simulink model "EvitarObstaculo"  (R2023b)
settings: Solver=FixedStepAuto  StartTime=0.0  StopTime=100  FixedStep=Ts  RelTol=1e-3
values from neighbouring files (symbols this model uses):
  obsx = 2    [TryOut.m]
  obsy = 0.5    [TryOut.m]
  refx = 5    [TryOut.m]
  refy = 5    [TryOut.m]
  Ts = 100e-3    (= 0.1)    [TryOut.m]
undefined symbols (not defined in the file or in its folder): DiscIntNeverNeededParam, sigbuilder_block, th_0, x_0, y_0
libraries: fuzblock x1
settings Model: Creator=Francisco  LastModifiedBy=Francisco
settings DataIOCC: ReturnWorkspaceOutputs=off

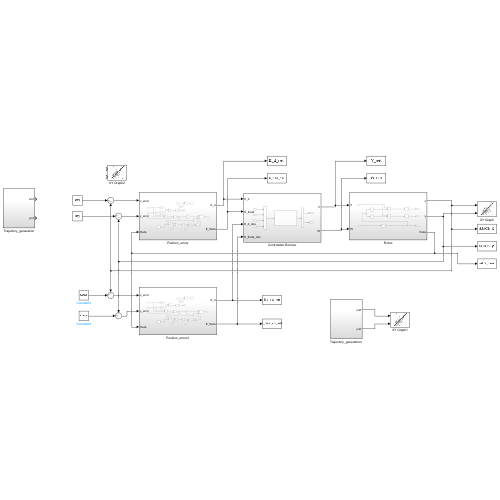
[thumbnail: Simulink's stored preview of the top-level diagram]
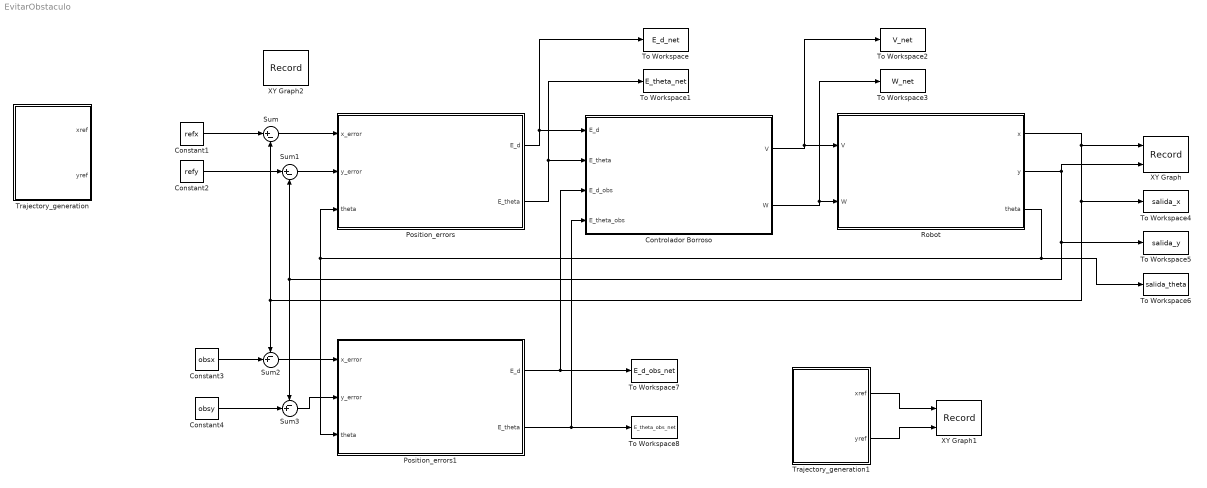
== system EvitarObstaculo ==
  Constant1 : Constant  Value=refx
  Constant2 : Constant  Value=refy
  Constant3 : Constant  Value=obsx
  Constant4 : Constant  Value=obsy
  Controlador Borroso : Subsystem
  Position_errors : Subsystem
  Position_errors1 : Subsystem
  Robot : Subsystem
  Sum : Sum  Inputs=|+-
  Sum1 : Sum  Inputs=|+-
  Sum2 : Sum  Inputs=-+|
  Sum3 : Sum  Inputs=-+|
  To Workspace : ToWorkspace  VariableName=E_d_net  SaveFormat=Structure With Time  SampleTime=-1
  To Workspace1 : ToWorkspace  VariableName=E_theta_net  SaveFormat=Structure With Time  SampleTime=-1
  To Workspace2 : ToWorkspace  VariableName=V_net  SaveFormat=Structure With Time  SampleTime=-1
  To Workspace3 : ToWorkspace  VariableName=W_net  SaveFormat=Structure With Time  SampleTime=-1
  To Workspace4 : ToWorkspace  VariableName=salida_x  SaveFormat=Structure With Time  SampleTime=-1
  To Workspace5 : ToWorkspace  VariableName=salida_y  SaveFormat=Structure With Time  SampleTime=-1
  To Workspace6 : ToWorkspace  VariableName=salida_theta  SaveFormat=Structure With Time  SampleTime=-1
  To Workspace7 : ToWorkspace  VariableName=E_d_obs_net  SaveFormat=Structure With Time  SampleTime=-1
  To Workspace8 : ToWorkspace  VariableName=E_theta_obs_net  SaveFormat=Structure With Time  SampleTime=-1
  Trajectory_generation : Subsystem
  Trajectory_generation1 : Subsystem
  XY Graph : Record  FileSettingsInternal="{\"entries\":[{\"content\":{\"excelSettings\":{\"content\":{},\"type\":\"Streamout.ExcelSettings\"}},\"type\":\"Streamout.FileSettingStorage\",\"uuid\":\"\"}],\"packageUris\":[\"http:\\/\\/schema.mathworks.com\\/mf0\\/streamout_blocks\\/R2020a\"],\"version\":\"1.0\"}"  Layout=[1 1]  SignalsInternal="{\"entries\":[{\"content\":{\"signals\":[{\"content\":{\"blockPath\":[],\"dimensions\":[1],\"domain\":\"\",\"lineColor\":\"#0072bd\",\"plots\":[1],\"port\":1,\"sid\":[\"\"],\"signalID\":8880,\"signalName\":\"Robot:1\"},\"type\":\"RecordBlkView.Signal\",\"uuid\":\"\"},{\"content\":{\"blockPath\":[],\"dimensions\":[1],\"domain\":\"\",\"lineColor\":\"#d95319\",\"plots\":[1],\"port\":2,\"sid\":[\"\"],\"signalID\":8884,\"signalName\":\"Robot:2\"},\"type\":\"RecordBlkView.Signal\",\"uuid\":\"\"}]},\"type\":\"RecordBlkView.InputSignals\",\"uuid\":\"\"}],\"packageUris\":[\"http:\\/\\/schema.mathworks.com\\/mf0\\/streamout_blocks\\/R2020a\"],\"version\":\"1.0\"}"  VisualizationBindings="{\"xyplotplugin\":{\"info\":[{\"series\":[{\"bindingParametersList\":[{\"parameter\":\"X-Axis\",\"signalID\":8880,\"signalName\":\"Robot:1\"},{\"parameter\":\"Y-Axis\",\"signalID\":8884,\"signalName\":\"Robot:2\"}],\"seriesID\":59230}],\"subplotID\":1}]}}"  CompatibilityTag=XY
  XY Graph1 : Record  FileSettingsInternal="{\"entries\":[{\"content\":{\"excelSettings\":{\"content\":{},\"type\":\"Streamout.ExcelSettings\"}},\"type\":\"Streamout.FileSettingStorage\",\"uuid\":\"\"}],\"packageUris\":[\"http:\\/\\/schema.mathworks.com\\/mf0\\/streamout_blocks\\/R2020a\"],\"version\":\"1.0\"}"  Layout=[1 1]  SignalsInternal="{\"entries\":[{\"content\":{\"signals\":[{\"content\":{\"blockPath\":[],\"dimensions\":[1],\"domain\":\"\",\"lineColor\":\"#b746ff\",\"plots\":[1],\"port\":1,\"sid\":[\"\"],\"signalID\":8932,\"signalName\":\"Trajectory_generation1:1\"},\"type\":\"RecordBlkView.Signal\",\"uuid\":\"\"},{\"content\":{\"blockPath\":[],\"dimensions\":[1],\"domain\":\"\",\"lineColor\":\"#64d413\",\"plots\":[1],\"port\":2,\"sid\":[\"\"],\"signalID\":8936,\"signalName\":\"Trajectory_generation1:2\"},\"type\":\"RecordBlkView.Signal\",\"uuid\":\"\"}]},\"type\":\"RecordBlkView.InputSignals\",\"uuid\":\"\"}],\"packageUris\":[\"http:\\/\\/schema.mathworks.com\\/mf0\\/streamout_blocks\\/R2020a\"],\"version\":\"1.0\"}"  VisualizationBindings="{\"xyplotplugin\":{\"info\":[{\"series\":[{\"bindingParametersList\":[{\"parameter\":\"X-Axis\",\"signalID\":8932,\"signalName\":\"Trajectory_generation1:1\"},{\"parameter\":\"Y-Axis\",\"signalID\":8936,\"signalName\":\"Trajectory_generation1:2\"}],\"seriesID\":46973}],\"subplotID\":1}]}}"  CompatibilityTag=XY
  XY Graph2 : Record  FileSettingsInternal="{\"entries\":[{\"content\":{\"excelSettings\":{\"content\":{},\"type\":\"Streamout.ExcelSettings\"}},\"type\":\"Streamout.FileSettingStorage\",\"uuid\":\"\"}],\"packageUris\":[\"http:\\/\\/schema.mathworks.com\\/mf0\\/streamout_blocks\\/R2020a\"],\"version\":\"1.0\"}"  Layout=[1 1]  SignalsInternal="{\"entries\":[{\"content\":{\"signals\":[{\"content\":{\"blockPath\":[],\"dimensions\":[1],\"domain\":\"\",\"lineColor\":\"#b746ff\",\"plots\":[1],\"port\":1,\"sid\":[\"\"],\"signalID\":8888,\"signalName\":\"Trajectory_generation:1\"},\"type\":\"RecordBlkView.Signal\",\"uuid\":\"\"},{\"content\":{\"blockPath\":[],\"dimensions\":[1],\"domain\":\"\",\"lineColor\":\"#64d413\",\"plots\":[1],\"port\":2,\"sid\":[\"\"],\"signalID\":8892,\"signalName\":\"Trajectory_generation:2\"},\"type\":\"RecordBlkView.Signal\",\"uuid\":\"\"}]},\"type\":\"RecordBlkView.InputSignals\",\"uuid\":\"\"}],\"packageUris\":[\"http:\\/\\/schema.mathworks.com\\/mf0\\/streamout_blocks\\/R2020a\"],\"version\":\"1.0\"}"  VisualizationBindings="{\"xyplotplugin\":{\"info\":[{\"series\":[{\"bindingParametersList\":[{\"parameter\":\"X-Axis\",\"signalID\":8888,\"signalName\":\"Trajectory_generation:1\"},{\"parameter\":\"Y-Axis\",\"signalID\":8892,\"signalName\":\"Trajectory_generation:2\"}],\"seriesID\":2748}],\"subplotID\":1}]}}"  CompatibilityTag=XY
  wires:
  Robot/3(theta) -> To Workspace6/1, Position_errors1/3(theta), Position_errors/3(theta)
  Position_errors/2(E_theta) -> Controlador Borroso/2(E_theta), To Workspace1/1
  Robot/1(x) -> XY Graph/1, To Workspace4/1, Sum2/1, Sum/2
  Controlador Borroso/1(V) -> To Workspace2/1, Robot/1(V)
  Controlador Borroso/2(W) -> To Workspace3/1, Robot/2(W)
  Position_errors/1(E_d) -> Controlador Borroso/1(E_d), To Workspace/1
  Sum/1 -> Position_errors/1(x_error)
  Sum1/1 -> Position_errors/2(y_error)
  Robot/2(y) -> XY Graph/2, Sum3/1, Sum1/2, To Workspace5/1
  Trajectory_generation1/2(yref) -> XY Graph1/2
  Trajectory_generation1/1(xref) -> XY Graph1/1
  Position_errors1/2(E_theta) -> Controlador Borroso/4(E_theta_obs), To Workspace8/1
  Position_errors1/1(E_d) -> Controlador Borroso/3(E_d_obs), To Workspace7/1
  Constant3/1 -> Sum2/2
  Constant4/1 -> Sum3/2
  Sum2/1 -> Position_errors1/1(x_error)
  Sum3/1 -> Position_errors1/2(y_error)
  Constant1/1 -> Sum/1
  Constant2/1 -> Sum1/1

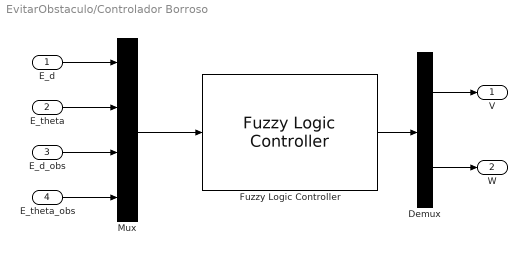
== system EvitarObstaculo/Controlador Borroso ==
  E_d : Inport
  E_theta : Inport  Port=2
  E_d_obs : Inport  Port=3
  E_theta_obs : Inport  Port=4
  Demux : Demux  Outputs=2
  Fuzzy Logic Controller : fuzblock/Fuzzy Logic  Controller  FIS='EvitarObstaculo.fis'  OutputSampleNumber=101  DataType=double  FuzzifiedInputs=off  RuleFiringStrengths=off  RuleOutputs=off  AggregatedOutputs=off  SimulateUsing=Interpreted execution  OutOfRangeInputValueMessage=warning  NoRuleFiredMessage=warning  EmptyOutputFuzzySetMessage=warning
  Mux : Mux
  V : Outport
  W : Outport  Port=2
  wires:
  Fuzzy Logic Controller/1 -> Demux/1
  Demux/1 -> V/1
  Demux/2 -> W/1
  E_theta_obs/1 -> Mux/4
  E_theta/1 -> Mux/2
  E_d_obs/1 -> Mux/3
  E_d/1 -> Mux/1
  Mux/1 -> Fuzzy Logic Controller/1

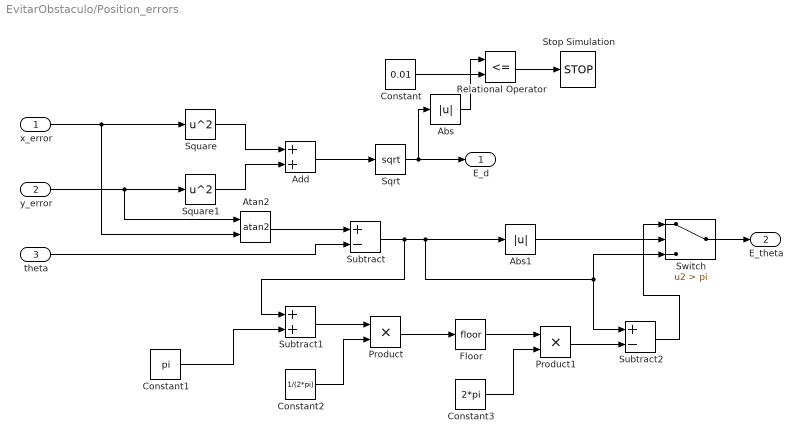
== system EvitarObstaculo/Position_errors ==
  x_error : Inport
  y_error : Inport  Port=2
  theta : Inport  Port=3
  Abs : Abs  SaturateOnIntegerOverflow=off
  Abs1 : Abs  SaturateOnIntegerOverflow=off
  Add : Sum
  Atan2 : Trigonometry  Operator=atan2
  Constant : Constant  Value=0.01
  Constant1 : Constant  Value=pi
  Constant2 : Constant  Value=1/(2*pi)
  Constant3 : Constant  Value=2*pi
  Floor : Rounding
  Product : Product
  Product1 : Product
  Relational Operator : RelationalOperator  Operator=<=  OutDataTypeStr=boolean  RndMeth=Simplest  InputSameDT=off
  Sqrt : Sqrt
  Square : Math  Operator=square
  Square1 : Math  Operator=square
  Stop Simulation : Stop
  Subtract : Sum  Inputs=+-
  Subtract1 : Sum
  Subtract2 : Sum  Inputs=+-
  Switch : Switch  Criteria=u2 > Threshold  Threshold=pi  SaturateOnIntegerOverflow=off  InputSameDT=off
  E_d : Outport
  E_theta : Outport  Port=2
  wires:
  x_error/1 -> Square/1, Atan2/2
  y_error/1 -> Atan2/1, Square1/1
  Square/1 -> Add/1
  Square1/1 -> Add/2
  Add/1 -> Sqrt/1
  Sqrt/1 -> E_d/1, Abs/1
  theta/1 -> Subtract/2
  Atan2/1 -> Subtract/1
  Constant/1 -> Relational Operator/2
  Abs/1 -> Relational Operator/1
  Switch/1 -> E_theta/1
  Subtract/1 -> Subtract1/1, Abs1/1, Switch/3, Subtract2/1
  Abs1/1 -> Switch/2
  Constant1/1 -> Subtract1/2
  Subtract1/1 -> Product/1
  Constant2/1 -> Product/2
  Product/1 -> Floor/1
  Floor/1 -> Product1/1
  Constant3/1 -> Product1/2
  Product1/1 -> Subtract2/2
  Subtract2/1 -> Switch/1
  Relational Operator/1 -> Stop Simulation/1

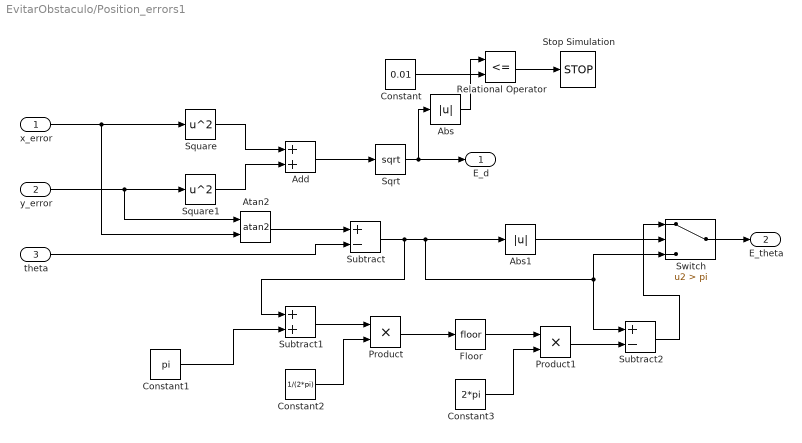
== system EvitarObstaculo/Position_errors1 ==
  x_error : Inport
  y_error : Inport  Port=2
  theta : Inport  Port=3
  Abs : Abs  SaturateOnIntegerOverflow=off
  Abs1 : Abs  SaturateOnIntegerOverflow=off
  Add : Sum
  Atan2 : Trigonometry  Operator=atan2
  Constant : Constant  Value=0.01
  Constant1 : Constant  Value=pi
  Constant2 : Constant  Value=1/(2*pi)
  Constant3 : Constant  Value=2*pi
  Floor : Rounding
  Product : Product
  Product1 : Product
  Relational Operator : RelationalOperator  Operator=<=  OutDataTypeStr=boolean  RndMeth=Simplest  InputSameDT=off
  Sqrt : Sqrt
  Square : Math  Operator=square
  Square1 : Math  Operator=square
  Stop Simulation : Stop
  Subtract : Sum  Inputs=+-
  Subtract1 : Sum
  Subtract2 : Sum  Inputs=+-
  Switch : Switch  Criteria=u2 > Threshold  Threshold=pi  SaturateOnIntegerOverflow=off  InputSameDT=off
  E_d : Outport
  E_theta : Outport  Port=2
  wires:
  x_error/1 -> Square/1, Atan2/2
  y_error/1 -> Atan2/1, Square1/1
  Square/1 -> Add/1
  Square1/1 -> Add/2
  Add/1 -> Sqrt/1
  Sqrt/1 -> E_d/1, Abs/1
  theta/1 -> Subtract/2
  Atan2/1 -> Subtract/1
  Relational Operator/1 -> Stop Simulation/1
  Constant/1 -> Relational Operator/2
  Abs/1 -> Relational Operator/1
  Switch/1 -> E_theta/1
  Subtract/1 -> Subtract1/1, Abs1/1, Switch/3, Subtract2/1
  Abs1/1 -> Switch/2
  Constant1/1 -> Subtract1/2
  Subtract1/1 -> Product/1
  Constant2/1 -> Product/2
  Product/1 -> Floor/1
  Floor/1 -> Product1/1
  Constant3/1 -> Product1/2
  Product1/1 -> Subtract2/2
  Subtract2/1 -> Switch/1

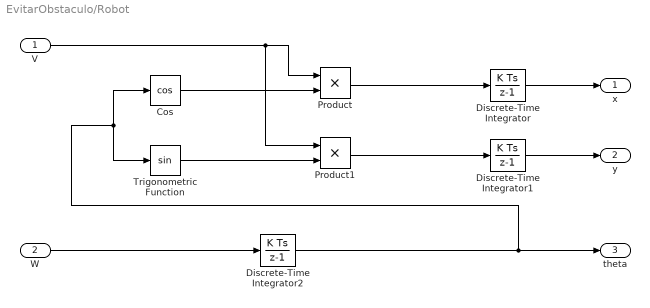
== system EvitarObstaculo/Robot ==
  V : Inport
  W : Inport  Port=2
  Cos : Trigonometry  Operator=cos
  Discrete-Time Integrator : DiscreteIntegrator  SampleTime=-1  ICPrevOutput=DiscIntNeverNeededParam  ICPrevScaledInput=DiscIntNeverNeededParam
  Discrete-Time Integrator1 : DiscreteIntegrator  SampleTime=-1  ICPrevOutput=DiscIntNeverNeededParam  ICPrevScaledInput=DiscIntNeverNeededParam
  Discrete-Time Integrator2 : DiscreteIntegrator  SampleTime=-1  ICPrevOutput=DiscIntNeverNeededParam  ICPrevScaledInput=DiscIntNeverNeededParam
  Product : Product
  Product1 : Product
  Trigonometric Function : Trigonometry
  x : Outport
  y : Outport  Port=2
  theta : Outport  Port=3
  wires:
  Discrete-Time Integrator2/1 -> theta/1, Trigonometric Function/1, Cos/1
  Product/1 -> Discrete-Time Integrator/1
  V/1 -> Product1/1, Product/1
  Discrete-Time Integrator1/1 -> y/1
  Trigonometric Function/1 -> Product1/2
  Product1/1 -> Discrete-Time Integrator1/1
  Cos/1 -> Product/2
  W/1 -> Discrete-Time Integrator2/1
  Discrete-Time Integrator/1 -> x/1

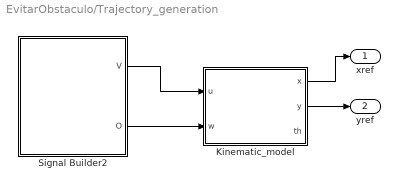
== system EvitarObstaculo/Trajectory_generation ==
  Kinematic_model : Subsystem
  Signal Builder2 : Subsystem  Tag=STV Subsys  LoadFcn=sigbuilder_block('load');  StartFcn=sigbuilder_block('start');  StopFcn=sigbuilder_block('stop');  ClipboardFcn=sigbuilder_block('clipboard');  mask(Sigbuilder block){tuvar=[0:10]}
      mask help: Sigbuilder GUI
      mask init:
      | if ~strcmp(get_param(bdroot(gcbh),'SimulationStatus'),'stopped') tuvar = sigbuilder_block('maskInit'); end
      settings: CopyFcn=sigbuilder_block('copy');  DeleteFcn=sigbuilder_block('delete');  ModelCloseFcn=sigbuilder_block('modelClose');  PreSaveFcn=sigbuilder_block('preSave');  PauseFcn=sigbuilder_block('pause')  ContinueFcn=sigbuilder_block('continue')  NameChangeFcn=sigbuilder_block('namechange');  OpenFcn=sigbuilder_block('open',[60 45 534.4 467.25 ]);  CloseFcn=sigbuilder_block('close');
      mask Display: plot(0, 0, 100, 100,[2, 2, 32, 32, 2], [68, 8, 8, 68, 68],[32, 2], [38, 38], [32, 19, 2],[53, 60, 44], [32, 17, 17, 2],[16, 16, 31, 31]);txt = getActiveGroup(gcbh);text(2, 100, txt,'verticalAlignment', 'top');
  xref : Outport  VectorParamsAs1DForOutWhenUnconnected=off
  yref : Outport  Port=2  VectorParamsAs1DForOutWhenUnconnected=off
  wires:
  Signal Builder2/1(V) -> Kinematic_model/1(u)
  Signal Builder2/2(O) -> Kinematic_model/2(w)
  Kinematic_model/1(x) -> xref/1
  Kinematic_model/2(y) -> yref/1

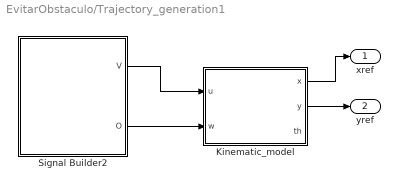
== system EvitarObstaculo/Trajectory_generation1 ==
  Kinematic_model : Subsystem
  Signal Builder2 : Subsystem  Tag=STV Subsys  LoadFcn=sigbuilder_block('load');  StartFcn=sigbuilder_block('start');  StopFcn=sigbuilder_block('stop');  ClipboardFcn=sigbuilder_block('clipboard');  mask(Sigbuilder block){tuvar=[0:10]}
      mask help: Sigbuilder GUI
      mask init:
      | if ~strcmp(get_param(bdroot(gcbh),'SimulationStatus'),'stopped') tuvar = sigbuilder_block('maskInit'); end
      settings: CopyFcn=sigbuilder_block('copy');  DeleteFcn=sigbuilder_block('delete');  ModelCloseFcn=sigbuilder_block('modelClose');  PreSaveFcn=sigbuilder_block('preSave');  PauseFcn=sigbuilder_block('pause')  ContinueFcn=sigbuilder_block('continue')  NameChangeFcn=sigbuilder_block('namechange');  OpenFcn=sigbuilder_block('open',[60 45 534.4 467.25 ]);  CloseFcn=sigbuilder_block('close');
      mask Display: plot(0, 0, 100, 100,[2, 2, 32, 32, 2], [68, 8, 8, 68, 68],[32, 2], [38, 38], [32, 19, 2],[53, 60, 44], [32, 17, 17, 2],[16, 16, 31, 31]);txt = getActiveGroup(gcbh);text(2, 100, txt,'verticalAlignment', 'top');
  xref : Outport  VectorParamsAs1DForOutWhenUnconnected=off
  yref : Outport  Port=2  VectorParamsAs1DForOutWhenUnconnected=off
  wires:
  Signal Builder2/1(V) -> Kinematic_model/1(u)
  Signal Builder2/2(O) -> Kinematic_model/2(w)
  Kinematic_model/1(x) -> xref/1
  Kinematic_model/2(y) -> yref/1

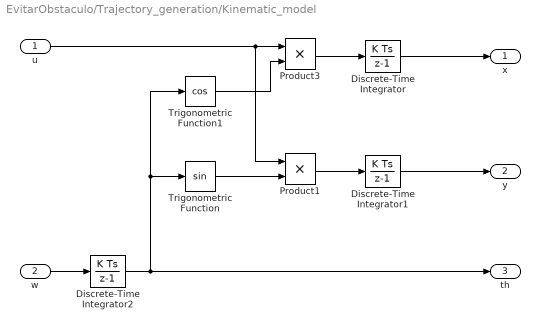
== system EvitarObstaculo/Trajectory_generation/Kinematic_model ==
  u : Inport
  w : Inport  Port=2
  Discrete-Time Integrator : DiscreteIntegrator  InitialCondition=x_0  SampleTime=Ts  ICPrevOutput=DiscIntNeverNeededParam  ICPrevScaledInput=DiscIntNeverNeededParam
  Discrete-Time Integrator1 : DiscreteIntegrator  InitialCondition=y_0  SampleTime=Ts  ICPrevOutput=DiscIntNeverNeededParam  ICPrevScaledInput=DiscIntNeverNeededParam
  Discrete-Time Integrator2 : DiscreteIntegrator  InitialCondition=th_0  SampleTime=Ts  ICPrevOutput=DiscIntNeverNeededParam  ICPrevScaledInput=DiscIntNeverNeededParam
  Product1 : Product
  Product3 : Product
  Trigonometric Function : Trigonometry
  Trigonometric Function1 : Trigonometry  Operator=cos
  x : Outport  VectorParamsAs1DForOutWhenUnconnected=off
  y : Outport  Port=2  VectorParamsAs1DForOutWhenUnconnected=off
  th : Outport  Port=3  VectorParamsAs1DForOutWhenUnconnected=off
  wires:
  Discrete-Time Integrator2/1 -> Trigonometric Function1/1, Trigonometric Function/1, th/1
  Product1/1 -> Discrete-Time Integrator1/1
  Product3/1 -> Discrete-Time Integrator/1
  w/1 -> Discrete-Time Integrator2/1
  Trigonometric Function/1 -> Product1/2
  u/1 -> Product1/1, Product3/1
  Trigonometric Function1/1 -> Product3/2
  Discrete-Time Integrator1/1 -> y/1
  Discrete-Time Integrator/1 -> x/1

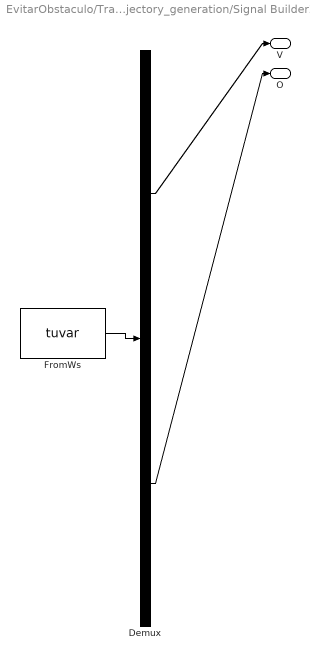
== system EvitarObstaculo/Trajectory_generation/Signal Builder2 ==
  Demux : Demux  Tag=STV Demux  Outputs=2
      settings: DisplayOption=none
  FromWs : FromWorkspace  Tag=STV FromWs  VariableName=tuvar
      SigBuilderData=|
      | common.afterFinalStr = 'Extrapolate'
      | common.sampleTime = '0'
      | dataSet.timeRange = [0 115]
      | dataSet.name = 'Group 1'
      | sbobj.Groups.Name = 'Group 1'
      | sbobj.Groups.Signals(1).Name = 'V'
      | sbobj.Groups.Signals(1).XData = [0 87 87 115]
      | sbobj.Groups.Signals(1).YData = [0.25 0.25 0 0]
      | sbobj.Groups.Signals(2).Name = 'O'
      | sbobj.Groups.Signals(2).XData = [0 12 12 30.849 30.849 55.981 55.981 74.83 74.83 99.962 115]
      | sbobj.Groups.Signals(2).YData = [0 0 0.25 0.25 -0.25 -0.25 0.25 0.25 0 0 0]
      | sbobj.Groups.TimeRange = [0 115]
  V : Outport  Tag=STV Outport  VectorParamsAs1DForOutWhenUnconnected=off
  O : Outport  Tag=STV Outport  Port=2  VectorParamsAs1DForOutWhenUnconnected=off
  wires:
  FromWs/1 -> Demux/1
  Demux/1 -> V/1
  Demux/2 -> O/1

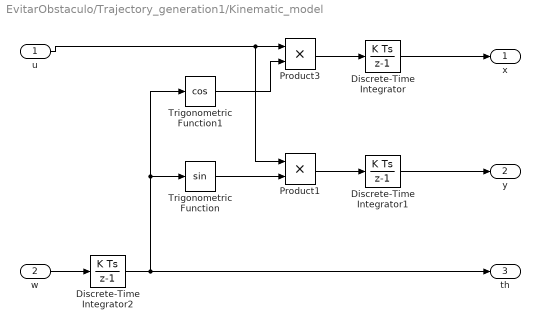
== system EvitarObstaculo/Trajectory_generation1/Kinematic_model ==
  u : Inport
  w : Inport  Port=2
  Discrete-Time Integrator : DiscreteIntegrator  InitialCondition=x_0  SampleTime=Ts  ICPrevOutput=DiscIntNeverNeededParam  ICPrevScaledInput=DiscIntNeverNeededParam
  Discrete-Time Integrator1 : DiscreteIntegrator  InitialCondition=y_0  SampleTime=Ts  ICPrevOutput=DiscIntNeverNeededParam  ICPrevScaledInput=DiscIntNeverNeededParam
  Discrete-Time Integrator2 : DiscreteIntegrator  InitialCondition=th_0  SampleTime=Ts  ICPrevOutput=DiscIntNeverNeededParam  ICPrevScaledInput=DiscIntNeverNeededParam
  Product1 : Product
  Product3 : Product
  Trigonometric Function : Trigonometry
  Trigonometric Function1 : Trigonometry  Operator=cos
  x : Outport  VectorParamsAs1DForOutWhenUnconnected=off
  y : Outport  Port=2  VectorParamsAs1DForOutWhenUnconnected=off
  th : Outport  Port=3  VectorParamsAs1DForOutWhenUnconnected=off
  wires:
  Discrete-Time Integrator2/1 -> Trigonometric Function1/1, Trigonometric Function/1, th/1
  Product1/1 -> Discrete-Time Integrator1/1
  Product3/1 -> Discrete-Time Integrator/1
  w/1 -> Discrete-Time Integrator2/1
  Trigonometric Function/1 -> Product1/2
  u/1 -> Product1/1, Product3/1
  Trigonometric Function1/1 -> Product3/2
  Discrete-Time Integrator1/1 -> y/1
  Discrete-Time Integrator/1 -> x/1

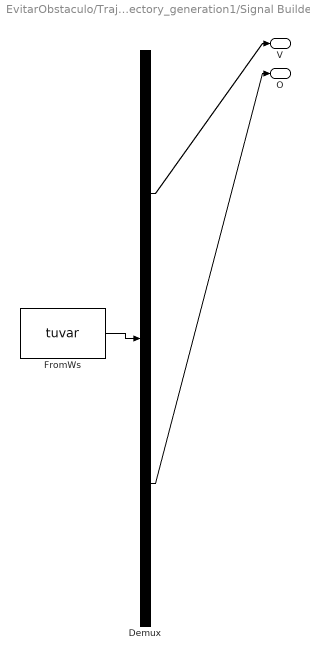
== system EvitarObstaculo/Trajectory_generation1/Signal Builder2 ==
  Demux : Demux  Tag=STV Demux  Outputs=2
      settings: DisplayOption=none
  FromWs : FromWorkspace  Tag=STV FromWs  VariableName=tuvar
      SigBuilderData=|
      | common.afterFinalStr = 'Extrapolate'
      | common.sampleTime = '0'
      | dataSet.timeRange = [0 115]
      | dataSet.name = 'Group 1'
      | sbobj.Groups.Name = 'Group 1'
      | sbobj.Groups.Signals(1).Name = 'V'
      | sbobj.Groups.Signals(1).XData = [0 87 87 115]
      | sbobj.Groups.Signals(1).YData = [0.25 0.25 0 0]
      | sbobj.Groups.Signals(2).Name = 'O'
      | sbobj.Groups.Signals(2).XData = [0 12 12 30.849 30.849 55.981 55.981 74.83 74.83 99.962 115]
      | sbobj.Groups.Signals(2).YData = [0 0 0.25 0.25 -0.25 -0.25 0.25 0.25 0 0 0]
      | sbobj.Groups.TimeRange = [0 115]
  V : Outport  Tag=STV Outport  VectorParamsAs1DForOutWhenUnconnected=off
  O : Outport  Tag=STV Outport  Port=2  VectorParamsAs1DForOutWhenUnconnected=off
  wires:
  FromWs/1 -> Demux/1
  Demux/1 -> V/1
  Demux/2 -> O/1
